simulink model "PD_control_with_adaptive_compensation"  (R2022a)
settings: Solver=FixedStepAuto  StartTime=0.0  StopTime=50  FixedStep=0.00001  RelTol=1e-3
settings Model: Creator=benja  LastModifiedBy=benja
settings DebuggingCC: UnderSpecifiedDimensionMsg=error

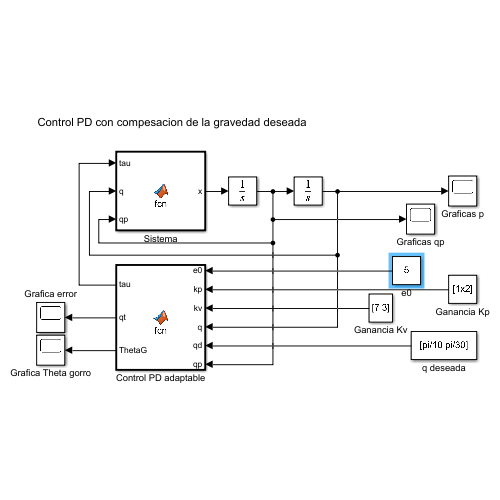
[thumbnail: Simulink's stored preview of the top-level diagram]
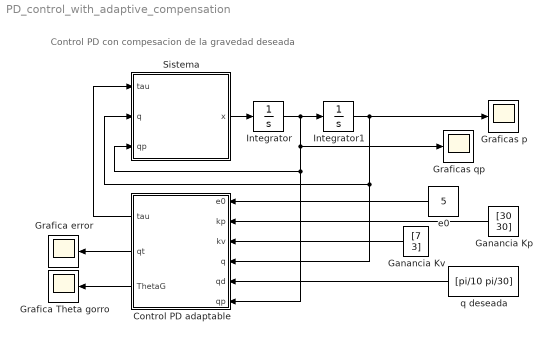
== system PD_control_with_adaptive_compensation ==
  note: Control PD con compesacion de la gravedad deseada
  Control PD adaptable : MATLAB Function  TreatAsAtomicUnit=on
  Ganancia Kp : Constant  Value=[30 30]
  Ganancia Kv : Constant  Value=[7 3]
  Grafica Theta gorro : Scope
  Grafica error : Scope
  Graficas p : Scope
  Graficas qp : Scope
  Integrator : Integrator  InitialCondition=[0 0]
  Integrator1 : Integrator  InitialCondition=[0 0]
  Sistema : MATLAB Function  TreatAsAtomicUnit=on
  e0 : Constant  Value=5
  q deseada : Constant  Value=[pi/10 pi/30]
  wires:
  Integrator/1 -> Control PD adaptable/6(qp), Sistema/3(qp), Graficas qp/1, Integrator1/1
  q deseada/1 -> Control PD adaptable/5(qd)
  Ganancia Kv/1 -> Control PD adaptable/3(kv)
  Ganancia Kp/1 -> Control PD adaptable/2(kp)
  e0/1 -> Control PD adaptable/1(e0)
  Sistema/1(x) -> Integrator/1
  Integrator1/1 -> Graficas p/1, Control PD adaptable/4(q), Sistema/2(q)
  Control PD adaptable/1(tau) -> Sistema/1(tau)
  Control PD adaptable/2(qt) -> Grafica error/1
  Control PD adaptable/3(ThetaG) -> Grafica Theta gorro/1

== matlab function PD_control_with_adaptive_compensation/Control PD adaptable ==
  settings: updateMethod=DISCRETE
  data: e0 input; tau output; kp input; kv input; q input; qd input; qp input; qt output; ThetaG output
function [tau, qt, ThetaG] = fcn(e0,kp, kv, q, qd, qp)
persistent int0t1
persistent int0t2

l1 = 0.26;
l2 = 0.26;
lc1 = 0.0983;
lc2 = 0.0229;
m1 = 6.5225;
m2 = 2.0458;
I1 = 0.1213;
I2 = 0.0116;
g = 9.81;

intt1 = 0;
intt2 = 0;

qt1 = qd(1) - q(1); 
qt2 = qd(2) - q(2);
qt = [qt1 qt2];

Gama = [500 10];

if isempty(int0t1)
    int0t1 = 0;
end

if isempty(int0t2)
    int0t2 = 0;
end

ThetaG0 = [0 0];

intt1 = ((e0/(1+norm(qt)))*qt(1))-qp(1);
intt2 = ((e0/(1+norm(qt)))*qt(2))-qp(2);

int0t1 = int0t1 + intt1*0.00001;
int0t2 = int0t2 + intt2*0.00001;

int0t = [int0t1 int0t2];

ThetaG1 = Gama(1)*l1*g*sin(qd(1))*int0t(1) + ThetaG0(1);

ThetaG2 = Gama(2)*g*sin(qd(1)+qd(2))*int0t(1) + Gama(2)*g*sin(qd(1)+qd(2))*int0t(2) + ThetaG0(2);

ThetaG = [ThetaG1 ThetaG2];

tau1 = kp(1)*qt(1) - kv(1)*qp(1) + l1*g*sin(qd(1))*ThetaG(1) + g*sin(qd(1)+qd(2))*ThetaG(2) + m1*lc1*g*sin(qd(1));
tau2 = kp(2)*qt(2) - kv(2)*qp(2) + g*sin(qd(1)+qd(2))*ThetaG(2);


tau = [tau1 tau2]';

== matlab function PD_control_with_adaptive_compensation/Sistema ==
  data: tau input; q input; qp input; x output
function x  = fcn(tau, q, qp)

l1 = 0.26;
l2 = 0.26;
lc1 = 0.0983;
lc2 = 0.0229;
m1 = 6.5225;
m2 = 2.0458;
I1 = 0.1213;
I2 = 0.0116;
g = 9.81;

M11 = m1*lc1^2 + m2*(l1^2 + lc2^2 + 2*l1*lc2*cos(q(2))) + I1 + I2;
M12 = m2*(lc2^2 + l1*lc2*cos(q(2))) + I2;
M21 = m2*(lc2^2 + l1*lc2*cos(q(2))) + I2;
M22 = m2*lc2^2 + I2;

C11 = -m2*l1*lc2*sin(q(2))*qp(2);
C12 = -m2*l1*lc2*sin(q(2))*(qp(1)+qp(2));
C21 = m2*l1*lc2*sin(q(2))*qp(1);
C22 = 0;

g1 = (m1*lc1+m2*l1)*g*sin(q(1)) + m2*lc2*g*sin(q(1) + q(2));
g2 = m2*lc2*g*sin(q(1)+q(2));

M = [M11 M12;M21 M22];

C = [C11 C12;C21 C22];

g = [g1; g2];

part1 = (tau-C*qp-g);

x = [inv(M)*part1]';
